simulink model "QRT_sim"  (Simulink 7.7)
settings: Solver=ode45  StartTime=0.0  StopTime=10  RelTol=1e-3
libraries: simulink x4
settings Model: Creator=page365  LastModifiedBy=page365
settings SFSimCC: SimParseCustomCode=off

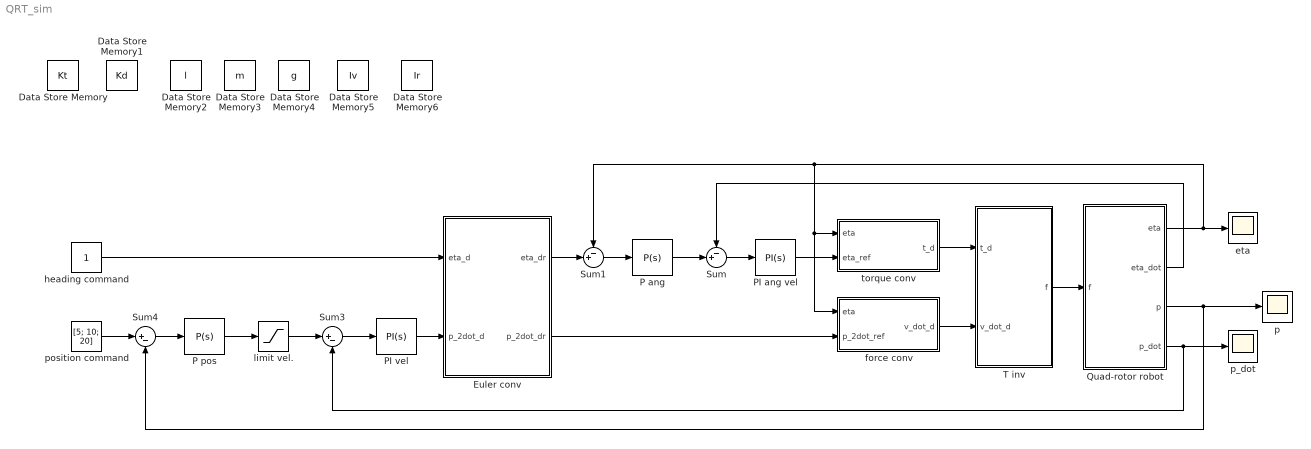
== system QRT_sim ==
  Data Store Memory : DataStoreMemory  DataStoreName=Kt  InitialValue=1  OutDataTypeStr=double
  Data Store Memory1 : DataStoreMemory  DataStoreName=Kd  InitialValue=0.2  OutDataTypeStr=double
  Data Store Memory2 : DataStoreMemory  DataStoreName=l  InitialValue=0.3  OutDataTypeStr=double
  Data Store Memory3 : DataStoreMemory  DataStoreName=m  InitialValue=2.2  OutDataTypeStr=double
  Data Store Memory4 : DataStoreMemory  DataStoreName=g  InitialValue=[0; 0; -9.81]  OutDataTypeStr=double
  Data Store Memory5 : DataStoreMemory  DataStoreName=Iv  InitialValue=[0.0170 0 0; 0 0.0170 0; 0 0 0.0230]  OutDataTypeStr=double
  Data Store Memory6 : DataStoreMemory  DataStoreName=Ir  InitialValue=[0.001 0 0; 0 0.001 0; 0 0 0.001]  OutDataTypeStr=double
  Euler conv : Stateflow chart  TreatAsAtomicUnit=on
  P ang : simulink/Continuous/PID Controller  SystemSampleTime=-1  Controller=P  TimeDomain=Continuous-time  SampleTime=1  IntegratorMethod=Forward Euler  FilterMethod=Forward Euler  Form=Parallel  P=5  I=0.00102076543610064  D=0  N=100  InitialConditionSource=internal  InitialConditionForIntegrator=0  InitialConditionForFilter=0  ExternalReset=none  LimitOutput=off  UpperSaturationLimit=inf  LowerSaturationLimit=-inf  LinearizeAsGain=off  AntiWindupMode=none  Kb=1  TrackingMode=off  Kt=1  PParamMin=[]  PParamMax=[]  IParamMin=[]  IParamMax=[]  DParamMin=[]  DParamMax=[]  NParamMin=[]  NParamMax=[]  KbParamMin=[]  KbParamMax=[]  KtParamMin=[]  KtParamMax=[]  POutMin=[]  POutMax=[]  IOutMin=[]  IOutMax=[]  DOutMin=[]  DOutMax=[]  NOutMin=[]  NOutMax=[]  KbOutMin=[]  KbOutMax=[]  KtOutMin=[]  KtOutMax=[]  IntegratorOutMin=[]  IntegratorOutMax=[]  FilterOutMin=[]  FilterOutMax=[]  SumOutMin=[]  SumOutMax=[]  SumI1OutMin=[]  SumI1OutMax=[]  SumI2OutMin=[]  SumI2OutMax=[]  SumI3OutMin=[]  SumI3OutMax=[]  SumDOutMin=[]  SumDOutMax=[]  SaturationOutMin=[]  SaturationOutMax=[]  IntegratorContinuousStateAttributes=''  IntegratorStateMustResolveToSignalObject=off  IntegratorRTWStateStorageClass=Auto  FilterContinuousStateAttributes=''  FilterStateMustResolveToSignalObject=off  FilterRTWStateStorageClass=Auto
  P pos : simulink/Continuous/PID Controller  SystemSampleTime=-1  Controller=P  TimeDomain=Continuous-time  SampleTime=1  IntegratorMethod=Forward Euler  FilterMethod=Forward Euler  Form=Parallel  P=1  I=0.00102076543610064  D=0  N=100  InitialConditionSource=internal  InitialConditionForIntegrator=0  InitialConditionForFilter=0  ExternalReset=none  LimitOutput=off  UpperSaturationLimit=inf  LowerSaturationLimit=-inf  LinearizeAsGain=off  AntiWindupMode=none  Kb=1  TrackingMode=off  Kt=1  PParamMin=[]  PParamMax=[]  IParamMin=[]  IParamMax=[]  DParamMin=[]  DParamMax=[]  NParamMin=[]  NParamMax=[]  KbParamMin=[]  KbParamMax=[]  KtParamMin=[]  KtParamMax=[]  POutMin=[]  POutMax=[]  IOutMin=[]  IOutMax=[]  DOutMin=[]  DOutMax=[]  NOutMin=[]  NOutMax=[]  KbOutMin=[]  KbOutMax=[]  KtOutMin=[]  KtOutMax=[]  IntegratorOutMin=[]  IntegratorOutMax=[]  FilterOutMin=[]  FilterOutMax=[]  SumOutMin=[]  SumOutMax=[]  SumI1OutMin=[]  SumI1OutMax=[]  SumI2OutMin=[]  SumI2OutMax=[]  SumI3OutMin=[]  SumI3OutMax=[]  SumDOutMin=[]  SumDOutMax=[]  SaturationOutMin=[]  SaturationOutMax=[]  IntegratorContinuousStateAttributes=''  IntegratorStateMustResolveToSignalObject=off  IntegratorRTWStateStorageClass=Auto  FilterContinuousStateAttributes=''  FilterStateMustResolveToSignalObject=off  FilterRTWStateStorageClass=Auto
  PI ang vel : simulink/Continuous/PID Controller  SystemSampleTime=-1  Controller=PI  TimeDomain=Continuous-time  SampleTime=1  IntegratorMethod=Forward Euler  FilterMethod=Forward Euler  Form=Parallel  P=20  I=100  D=0  N=100  InitialConditionSource=internal  InitialConditionForIntegrator=0  InitialConditionForFilter=0  ExternalReset=none  LimitOutput=off  UpperSaturationLimit=inf  LowerSaturationLimit=-inf  LinearizeAsGain=off  AntiWindupMode=none  Kb=1  TrackingMode=off  Kt=1  PParamMin=[]  PParamMax=[]  IParamMin=[]  IParamMax=[]  DParamMin=[]  DParamMax=[]  NParamMin=[]  NParamMax=[]  KbParamMin=[]  KbParamMax=[]  KtParamMin=[]  KtParamMax=[]  POutMin=[]  POutMax=[]  IOutMin=[]  IOutMax=[]  DOutMin=[]  DOutMax=[]  NOutMin=[]  NOutMax=[]  KbOutMin=[]  KbOutMax=[]  KtOutMin=[]  KtOutMax=[]  IntegratorOutMin=[]  IntegratorOutMax=[]  FilterOutMin=[]  FilterOutMax=[]  SumOutMin=[]  SumOutMax=[]  SumI1OutMin=[]  SumI1OutMax=[]  SumI2OutMin=[]  SumI2OutMax=[]  SumI3OutMin=[]  SumI3OutMax=[]  SumDOutMin=[]  SumDOutMax=[]  SaturationOutMin=[]  SaturationOutMax=[]  IntegratorContinuousStateAttributes=''  IntegratorStateMustResolveToSignalObject=off  IntegratorRTWStateStorageClass=Auto  FilterContinuousStateAttributes=''  FilterStateMustResolveToSignalObject=off  FilterRTWStateStorageClass=Auto
  PI vel : simulink/Continuous/PID Controller  SystemSampleTime=-1  Controller=PI  TimeDomain=Continuous-time  SampleTime=1  IntegratorMethod=Forward Euler  FilterMethod=Forward Euler  Form=Parallel  P=2  I=0  D=0  N=100  InitialConditionSource=internal  InitialConditionForIntegrator=0  InitialConditionForFilter=0  ExternalReset=none  LimitOutput=off  UpperSaturationLimit=inf  LowerSaturationLimit=-inf  LinearizeAsGain=off  AntiWindupMode=none  Kb=1  TrackingMode=off  Kt=1  PParamMin=[]  PParamMax=[]  IParamMin=[]  IParamMax=[]  DParamMin=[]  DParamMax=[]  NParamMin=[]  NParamMax=[]  KbParamMin=[]  KbParamMax=[]  KtParamMin=[]  KtParamMax=[]  POutMin=[]  POutMax=[]  IOutMin=[]  IOutMax=[]  DOutMin=[]  DOutMax=[]  NOutMin=[]  NOutMax=[]  KbOutMin=[]  KbOutMax=[]  KtOutMin=[]  KtOutMax=[]  IntegratorOutMin=[]  IntegratorOutMax=[]  FilterOutMin=[]  FilterOutMax=[]  SumOutMin=[]  SumOutMax=[]  SumI1OutMin=[]  SumI1OutMax=[]  SumI2OutMin=[]  SumI2OutMax=[]  SumI3OutMin=[]  SumI3OutMax=[]  SumDOutMin=[]  SumDOutMax=[]  SaturationOutMin=[]  SaturationOutMax=[]  IntegratorContinuousStateAttributes=''  IntegratorStateMustResolveToSignalObject=off  IntegratorRTWStateStorageClass=Auto  FilterContinuousStateAttributes=''  FilterStateMustResolveToSignalObject=off  FilterRTWStateStorageClass=Auto
  Quad-rotor robot : Subsystem
  Sum : Sum  Inputs=-+|
  Sum1 : Sum  Inputs=-+|
  Sum3 : Sum  Inputs=|+-
  Sum4 : Sum  Inputs=|+-
  T inv : Stateflow chart  TreatAsAtomicUnit=on
  eta : Scope
      settings: TimeRange=10  YMin=-0.5  YMax=1.5
  force conv : Stateflow chart  TreatAsAtomicUnit=on
  heading command : Constant
  limit vel. : Saturate  UpperLimit=5  LowerLimit=-5
  p : Scope
      settings: TimeRange=10  YMax=25
  p_dot : Scope
      settings: TimeRange=10  YMin=-1  YMax=6  SaveName=ScopeData2
  position command : Constant  Value=[5; 10; 20]
  torque conv : Stateflow chart  TreatAsAtomicUnit=on
  wires:
  T inv/1(f) -> Quad-rotor robot/1(f)
  torque conv/1(t_d) -> T inv/1(t_d)
  force conv/1(v_dot_d) -> T inv/2(v_dot_d)
  Quad-rotor robot/2(eta_dot) -> Sum/1
  Quad-rotor robot/1(eta) -> force conv/1(eta), torque conv/1(eta), Sum1/1, eta/1
  Sum1/1 -> P ang/1
  Quad-rotor robot/4(p_dot) -> p_dot/1, Sum3/2
  PI ang vel/1 -> torque conv/2(eta_ref)
  Sum/1 -> PI ang vel/1
  P ang/1 -> Sum/2
  Euler conv/1(eta_dr) -> Sum1/2
  Sum4/1 -> P pos/1
  Sum3/1 -> PI vel/1
  position command/1 -> Sum4/1
  Euler conv/2(p_2dot_dr) -> force conv/2(p_2dot_ref)
  PI vel/1 -> Euler conv/2(p_2dot_d)
  heading command/1 -> Euler conv/1(eta_d)
  P pos/1 -> limit vel./1
  Quad-rotor robot/3(p) -> p/1, Sum4/2
  limit vel./1 -> Sum3/1

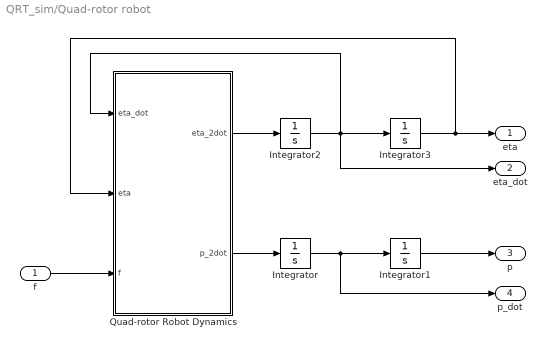
== system QRT_sim/Quad-rotor robot ==
  f : Inport
  Integrator{,1..3} (4 alike) : Integrator
  Quad-rotor Robot Dynamics : Stateflow chart  TreatAsAtomicUnit=on
  eta : Outport
  eta_dot : Outport  Port=2
  p : Outport  Port=3
  p_dot : Outport  Port=4
  wires:
  Integrator/1 -> Integrator1/1, p_dot/1
  Integrator1/1 -> p/1
  Quad-rotor Robot Dynamics/2(p_2dot) -> Integrator/1
  Quad-rotor Robot Dynamics/1(eta_2dot) -> Integrator2/1
  Integrator2/1 -> Integrator3/1, eta_dot/1, Quad-rotor Robot Dynamics/1(eta_dot)
  Integrator3/1 -> eta/1, Quad-rotor Robot Dynamics/2(eta)
  f/1 -> Quad-rotor Robot Dynamics/3(f)

== matlab function T inv ==
  data: t_d input double size=3; f output double size=4; v_dot_d input double size=1; Kd data_store_memory double size=1; l data_store_memory double size=1; m data_store_memory double size=1
function f = fcn(t_d, v_dot_d)

global Kd l m

r = Kd;

T = [1/m  1/m  1/m  1/m;
     0    -l   0    l;
     -l   0    l    0;
     r    -r   r    -r];

u = [v_dot_d(1,1); t_d(1,1); t_d(2,1); t_d(3,1)]; 
 
f = inv(T)*u;

% limits min and max force from rotor
% because motor can't make unlimited force
min_f = 0;
max_f = 10;

if (f(1,1) < min_f) f(1,1) = min_f; end
if (f(2,1) < min_f) f(2,1) = min_f; end
if (f(3,1) < min_f) f(3,1) = min_f; end
if (f(4,1) < min_f) f(4,1) = min_f; end

if (f(1,1) > max_f) f(1,1) = max_f; end
if (f(2,1) > max_f) f(2,1) = max_f; end
if (f(3,1) > max_f) f(3,1) = max_f; end
if (f(4,1) > max_f) f(4,1) = max_f; end

== matlab function Quad-rotor robot/Quad-rotor Robot Dynamics ==
  data: eta_dot input double size=3; eta_2dot output double size=3; eta input double size=3; p_2dot output double size=3; f input double size=4; Kt data_store_memory double; Kd data_store_memory double; l data_store_memory double; m data_store_memory double; g data_store_memory double; Iv data_store_memory double; Ir data_store_memory double
function [eta_2dot, p_2dot] = fcn(eta_dot, eta, f)

global Kt Kd l m g Iv Ir;
  
phi_dot = eta_dot(1,1);
theta_dot = eta_dot(2,1);
psi_dot = eta_dot(3,1);

sphi = sin(eta(1,1));
cphi = cos(eta(1,1));
stht = sin(eta(2,1));
ctht = cos(eta(2,1));
spsi = sin(eta(3,1));
cpsi = cos(eta(3,1));

R = [cpsi*ctht cpsi*stht*sphi-spsi*cphi cpsi*stht*cphi+spsi*sphi;	
     spsi*ctht spsi*stht*sphi+cpsi*cphi spsi*stht*cphi-cpsi*sphi;	
     -stht     ctht*sphi                ctht*cphi];

C = [1 0     -spsi;
     0 cphi  sphi*ctht;
     0 -sphi cphi*ctht];
 
C_dot = [0 0              -theta_dot*ctht;
         0 -phi_dot*sphi  phi_dot*cphi*ctht-theta_dot*sphi*stht;
         0 -phi_dot*cphi  -phi_dot*sphi*ctht-theta_dot*cphi*stht];

F1 = Kt*f(1,1);
F2 = Kt*f(2,1);
F3 = Kt*f(3,1);
F4 = Kt*f(4,1);
     
t1 = Kd*f(1,1);
t2 = Kd*f(2,1);
t3 = Kd*f(3,1);
t4 = Kd*f(4,1);
     
F = [0; 0; F1+F2+F3+F4];
Q = [l*(F4-F2); l*(F3-F1); t1-t2+t3-t4];
 
p_2dot = g + R*F/m;
eta_2dot = inv(Iv*C)*Q;

== matlab function torque conv ==
  data: eta input double size=3; eta_ref input double size=3; t_d output double size=3; Iv data_store_memory double size=3
function t_d = fcn(eta, eta_ref)

global Iv;

sphi = sin(eta(1,1));
cphi = cos(eta(1,1));
stht = sin(eta(2,1));
ctht = cos(eta(2,1));
spsi = sin(eta(3,1));
cpsi = cos(eta(3,1));

C = [1   0     -stht;
     0   cphi  sphi*ctht;
     0   -sphi cphi*ctht];

t_d = Iv*C*eta_ref;

== matlab function force conv ==
  data: eta input double size=3; p_2dot_ref input double size=1; v_dot_d output double size=1
function v_dot_d = fcn(eta, p_2dot_ref)

sphi = sin(eta(1,1));
cphi = cos(eta(1,1));
stht = sin(eta(2,1));
ctht = cos(eta(2,1));
spsi = sin(eta(3,1));
cpsi = cos(eta(3,1));

R = [cpsi*ctht cpsi*stht*sphi-spsi*cphi cpsi*stht*cphi+spsi*sphi;	
     spsi*ctht spsi*stht*sphi+cpsi*cphi spsi*stht*cphi-cpsi*sphi;	
     -stht     ctht*sphi                ctht*cphi];

u = [0; 0; p_2dot_ref(1,1)];
d = R'*u;

v_dot_d = d(3,1);

== matlab function Euler conv ==
  data: eta_d input double size=1; p_2dot_d input double size=3; eta_dr output double size=3; p_2dot_dr output double size=1
function [eta_dr, p_2dot_dr] = fcn(eta_d, p_2dot_d)
%#eml

psi_d = eta_d(1,1);

x_2dot_d = p_2dot_d(1,1);
y_2dot_d = p_2dot_d(2,1);
z_2dot_d = p_2dot_d(3,1) + 9.81;

d = sqrt(x_2dot_d*x_2dot_d + y_2dot_d*y_2dot_d + z_2dot_d*z_2dot_d);

if (-0.001 < d & d < 0.001)
    phi_d_ref = 0;
else
    phi_d_ref = asin((x_2dot_d*sin(psi_d) - y_2dot_d*cos(psi_d))/d);
end

theta_dr = atan2(x_2dot_d*cos(psi_d) + y_2dot_d*sin(psi_d), z_2dot_d);

min_ang = -pi/6;
max_ang =  pi/6;

if (phi_d_ref < min_ang) phi_d_ref = min_ang; end
if (phi_d_ref > max_ang) phi_d_ref = max_ang; end

if (theta_dr < min_ang) theta_dr = min_ang; end
if (theta_dr > max_ang) theta_dr = max_ang; end

eta_dr   = [phi_d_ref; theta_dr; psi_d];
p_2dot_dr = [z_2dot_d];
